simulink library "INT_StSys_AddCor"  (R2016b)
settings: Solver=VariableStepAuto  StartTime=0.0  StopTime=10.0  RelTol=1e-3
settings Model: Creator=zhoutinglin  LastModifiedBy=zhoutinglin

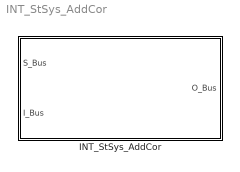
== system INT_StSys_AddCor ==
  INT_StSys_AddCor : Subsystem

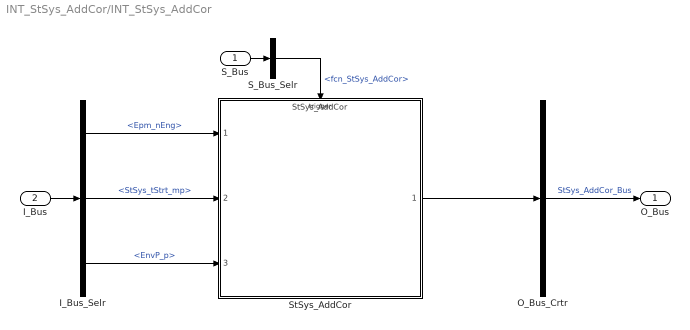
== system INT_StSys_AddCor/INT_StSys_AddCor ==
  S_Bus : Inport
  I_Bus : Inport  Port=2
  I_Bus_Selr : BusSelector  OutputSignals=Epm_nEng,StSys_tStrt_mp,EnvP_p
  O_Bus_Crtr : BusCreator  Inputs=1
  S_Bus_Selr : BusSelector  OutputSignals=fcn_StSys_AddCor
  StSys_AddCor : ModelReference  ModelNameDialog=StSys_AddCor  SimulationMode=Normal  ModelReferenceVersion=1.9  TriggerPortName=function  TriggerPortTriggerType=function-call  TriggerPortStatesWhenEnabling=held
  O_Bus : Outport
  wires:
  S_Bus_Selr/1 -> StSys_AddCor/Trigger  "<fcn_StSys_AddCor>"
  S_Bus/1 -> S_Bus_Selr/1
  I_Bus/1 -> I_Bus_Selr/1
  I_Bus_Selr/1 -> StSys_AddCor/1  "<Epm_nEng>"
  I_Bus_Selr/2 -> StSys_AddCor/2  "<StSys_tStrt_mp>"
  I_Bus_Selr/3 -> StSys_AddCor/3  "<EnvP_p>"
  O_Bus_Crtr/1 -> O_Bus/1  "StSys_AddCor_Bus"
  StSys_AddCor/1 -> O_Bus_Crtr/1
